simulink model "model_ROV_MPC_wLinFeed_NoTime"  (R2022b)
settings: Solver=VariableStepAuto  StartTime=0.0  StopTime=50  RelTol=1e-3
undefined symbols (not defined in the file): dt, magnitude, t0
libraries: realtime_pacer_lib x1, sim3dlib x1, uavsim3dlib x1
settings Model: Creator=anton  LastModifiedBy=anton

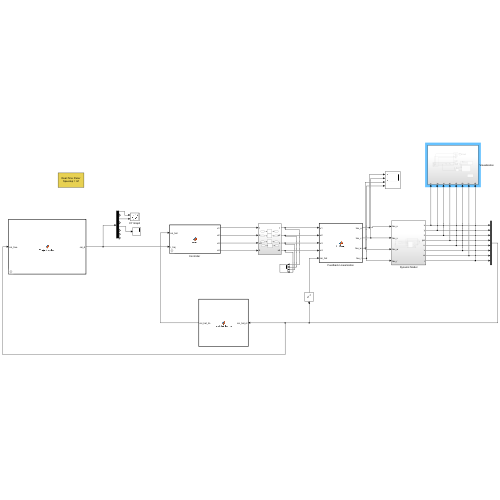
[thumbnail: Simulink's stored preview of the top-level diagram]
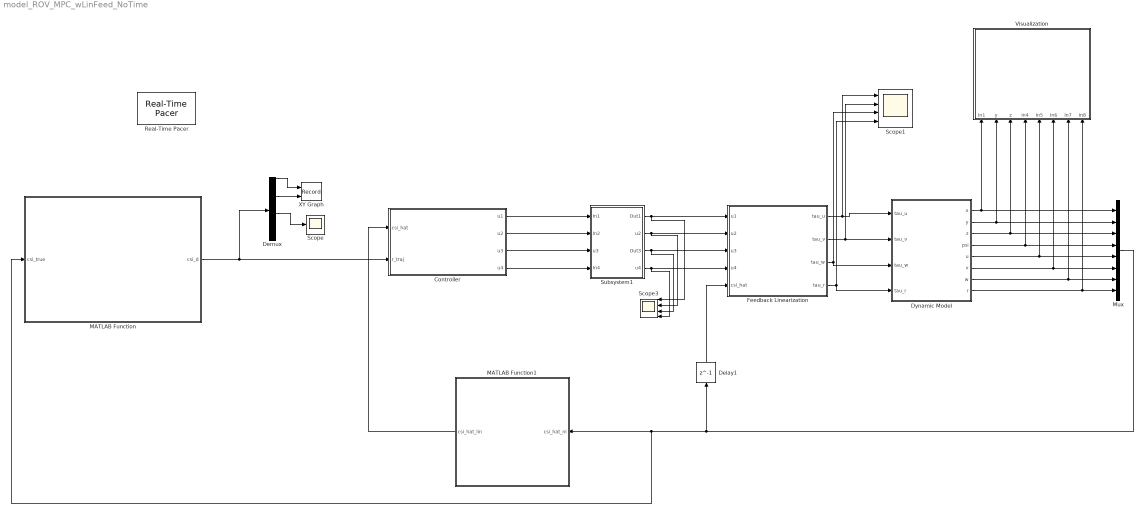
== system model_ROV_MPC_wLinFeed_NoTime ==
  "Controller " : MATLAB Function  TreatAsAtomicUnit=on  mask{dt=dt, t0=t0}
      mask prompts: dt "tempo di campionamento"; t0 "Start mission time"
  Delay1 : Delay  DelayLength=1  InitialCondition=[0 0 0 0 0 0 0 0]'  SampleTime=dt
  Demux : Demux  Outputs=8
  Dynamic Model : Subsystem
  Feedback Linearization : MATLAB Function  TreatAsAtomicUnit=on
  MATLAB Function : MATLAB Function  TreatAsAtomicUnit=on  mask{t0=t0}
      mask prompts: t0 "Tempo di partenza"
  MATLAB Function1 : MATLAB Function  TreatAsAtomicUnit=on
  Mux : Mux  Inputs=8
  Real-Time Pacer : realtime_pacer_lib/Real-Time Pacer  simTimePerRealTime=inf
  Scope : Scope
  Scope1 : Scope  NumInputPorts=4
  Scope3 : Scope  NumInputPorts=4
  Subsystem1 : Subsystem
  Visualization : Subsystem
  XY Graph : Record  FileSettingsInternal="{\"entries\":[{\"content\":{\"excelSettings\":{\"content\":{},\"type\":\"Streamout.ExcelSettings\"}},\"type\":\"Streamout.FileSettingStorage\",\"uuid\":\"\"}],\"packageUris\":[\"http:\\/\\/schema.mathworks.com\\/mf0\\/streamout_blocks\\/R2020a\"],\"version\":\"1.0\"}"  Layout=[1 1]  SignalsInternal="{\"entries\":[{\"content\":{\"signals\":[{\"content\":{\"blockPath\":[],\"channel\":[],\"dimensions\":[1,1],\"domain\":\"\",\"lineColor\":\"#a2142f\",\"plots\":[1],\"port\":1,\"sid\":[\"\"],\"signalID\":10914,\"signalName\":\"Demux:1\"},\"type\":\"RecordBlkView.Signal\",\"uuid\":\"\"},{\"content\":{\"blockPath\":[],\"channel\":[],\"dimensions\":[1,1],\"domain\":\"\",\"lineColor\":\"#139fff\",\"plots\":[1],\"port\":2,\"sid\":[\"\"],\"signalID\":10918,\"signalName\":\"Demux:3\"},\"type\":\"RecordBlkView.Signal\",\"uuid\":\"\"}]},\"type\":\"RecordBlkView.InputSignals\",\"uuid\":\"\"}],\"packageUris\":[\"http:\\/\\/schema.mathworks.com\\/mf0\\/streamout_blocks\\/R2020a\"],\"version\":\"1.0\"}"  VisualizationBindings="{\"xyplotplugin\":{\"info\":[{\"series\":[{\"bindingParametersList\":[{\"parameter\":\"X-Axis\",\"signalID\":10914,\"signalName\":\"Demux:1\"},{\"parameter\":\"Y-Axis\",\"signalID\":10918,\"signalName\":\"Demux:3\"}],\"seriesID\":62600}],\"subplotID\":1}]}}"  CompatibilityTag=XY
  wires:
  Subsystem1/2(u2) -> Feedback Linearization/2(u2), Scope3/2
  Subsystem1/3(Out3) -> Feedback Linearization/3(u3), Scope3/3
  Subsystem1/4(u4) -> Scope3/4, Feedback Linearization/4(u4)
  "Controller "/1(u1) -> Subsystem1/1(In1)
  "Controller "/2(u2) -> Subsystem1/2(In2)
  "Controller "/3(u3) -> Subsystem1/3(u3)
  "Controller "/4(u4) -> Subsystem1/4(In4)
  Subsystem1/1(Out1) -> Scope3/1, Feedback Linearization/1(u1)
  MATLAB Function1/1(csi_hat_lin) -> "Controller "/1(csi_hat)
  Dynamic Model/1(x) -> Mux/1, Visualization/1(In1)
  Dynamic Model/2(y) -> Mux/2, Visualization/2(y)
  Dynamic Model/3(z) -> Mux/3, Visualization/3(z)
  Dynamic Model/4(psi) -> Mux/4, Visualization/4(In4)
  Dynamic Model/5(u) -> Mux/5, Visualization/5(In5)
  Dynamic Model/6(v) -> Mux/6, Visualization/6(In6)
  Dynamic Model/7(w) -> Mux/7, Visualization/7(In7)
  Dynamic Model/8(r) -> Mux/8, Visualization/8(In8)
  Feedback Linearization/1(tau_u) -> Dynamic Model/1(tau_u), Scope1/1
  Feedback Linearization/2(tau_v) -> Scope1/2, Dynamic Model/2(tau_v)
  Feedback Linearization/3(tau_w) -> Dynamic Model/3(tau_w), Scope1/3
  Feedback Linearization/4(tau_r) -> Dynamic Model/4(tau_r), Scope1/4
  Mux/1 -> Delay1/1, MATLAB Function/1(csi_true), MATLAB Function1/1(csi_hat_nl)
  Delay1/1 -> Feedback Linearization/5(csi_hat)
  MATLAB Function/1(csi_d) -> Demux/1, "Controller "/2(r_traj)
  Demux/1 -> XY Graph/1
  Demux/3 -> XY Graph/2
  Demux/5 -> Scope/1

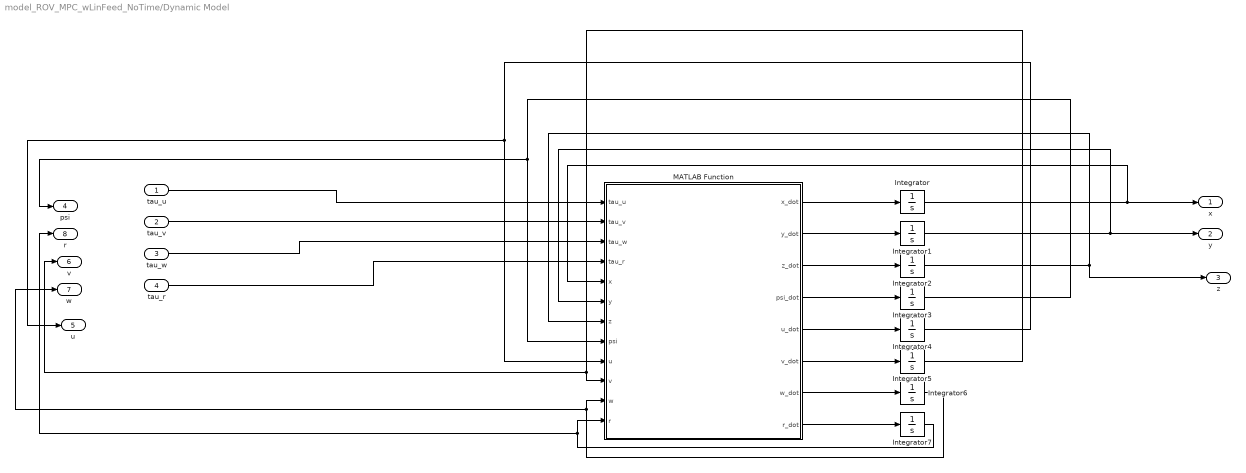
== system model_ROV_MPC_wLinFeed_NoTime/Dynamic Model ==
  tau_u : Inport
  tau_v : Inport  Port=2
  tau_w : Inport  Port=3
  tau_r : Inport  Port=4
  Integrator{,1..7} (8 alike) : Integrator
  MATLAB Function : MATLAB Function  TreatAsAtomicUnit=on
  x : Outport
  y : Outport  Port=2
  z : Outport  Port=3
  psi : Outport  Port=4
  u : Outport  Port=5
  v : Outport  Port=6
  w : Outport  Port=7
  r : Outport  Port=8
  wires:
  MATLAB Function/1(x_dot) -> Integrator/1
  Integrator3/1 -> psi/1, MATLAB Function/8(psi)
  MATLAB Function/6(v_dot) -> Integrator5/1
  MATLAB Function/4(psi_dot) -> Integrator3/1
  Integrator2/1 -> MATLAB Function/7(z), z/1
  Integrator4/1 -> u/1, MATLAB Function/9(u)
  Integrator6/1 -> w/1, MATLAB Function/11(w)
  Integrator7/1 -> r/1, MATLAB Function/12(r)
  MATLAB Function/5(u_dot) -> Integrator4/1
  MATLAB Function/7(w_dot) -> Integrator6/1
  tau_v/1 -> MATLAB Function/2(tau_v)
  MATLAB Function/8(r_dot) -> Integrator7/1
  tau_w/1 -> MATLAB Function/3(tau_w)
  MATLAB Function/3(z_dot) -> Integrator2/1
  Integrator1/1 -> y/1, MATLAB Function/6(y)
  Integrator5/1 -> v/1, MATLAB Function/10(v)
  tau_r/1 -> MATLAB Function/4(tau_r)
  Integrator/1 -> x/1, MATLAB Function/5(x)
  MATLAB Function/2(y_dot) -> Integrator1/1
  tau_u/1 -> MATLAB Function/1(tau_u)

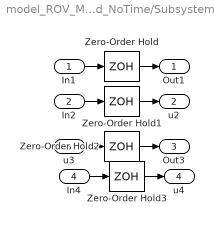
== system model_ROV_MPC_wLinFeed_NoTime/Subsystem1 ==
  In1 : Inport
  In2 : Inport  Port=2
  u3 : Inport  Port=3
  In4 : Inport  Port=4
  Zero-Order Hold{,1..3} (4 alike) : ZeroOrderHold  SampleTime=dt
  Out1 : Outport
  u2 : Outport  Port=2
  Out3 : Outport  Port=3
  u4 : Outport  Port=4
  wires:
  In1/1 -> Zero-Order Hold/1
  Zero-Order Hold/1 -> Out1/1
  In4/1 -> Zero-Order Hold3/1
  Zero-Order Hold1/1 -> u2/1
  Zero-Order Hold3/1 -> u4/1
  u3/1 -> Zero-Order Hold2/1
  In2/1 -> Zero-Order Hold1/1
  Zero-Order Hold2/1 -> Out3/1

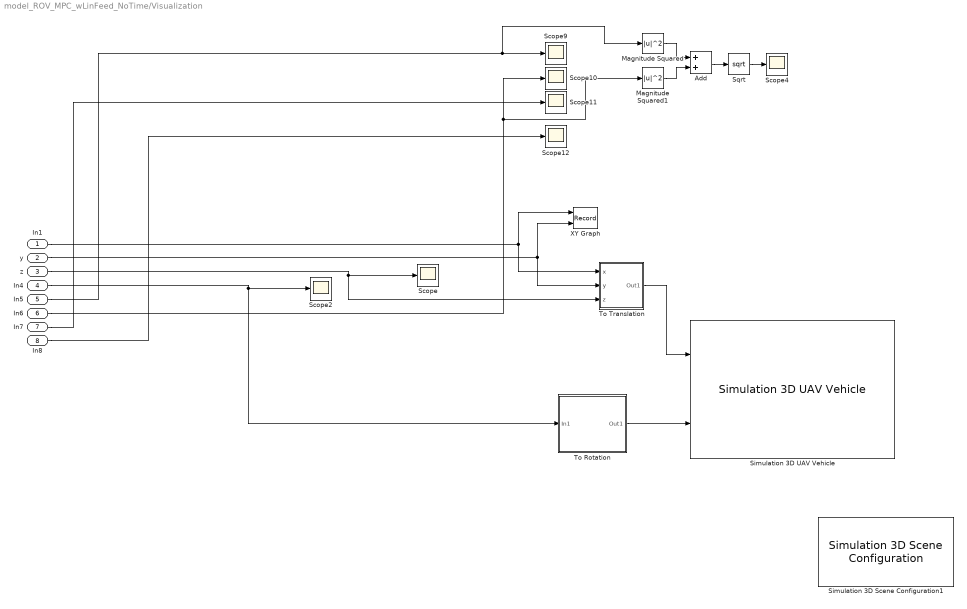
== system model_ROV_MPC_wLinFeed_NoTime/Visualization ==
  In1 : Inport
  y : Inport  Port=2
  z : Inport  Port=3
  In4 : Inport  Port=4
  In5 : Inport  Port=5
  In6 : Inport  Port=6
  In7 : Inport  Port=7
  In8 : Inport  Port=8
  Add : Sum
  Magnitude Squared : Math  Operator=magnitude^2
  Magnitude Squared1 : Math  Operator=magnitude^2
  Scope{,2,4,9..12} (7 alike) : Scope
  Simulation 3D Scene Configuration1 : sim3dlib/Simulation 3D Scene Configuration  Priority=0  ProjectFormat=Unreal Executable  SceneDesc=Empty scene  ProjectName=C:\Program Files\MATLAB\R2022b\toolbox\shared\sim3d_projects\automotive_project\UE4\WindowsNoEditor\VehicleSimulation.exe  ScenePath=/Game/Maps/HwStrght  EnableOpenDRIVE=off  vehTagList={'Scene Origin';'SimulinkVehicle1'}  vehTag=SimulinkVehicle1  OpVisEn=off  Ts=.02  EnableWindow=on  EnableRemoteAccess=off  EnableWeather=off  SunAltitude=40.0  SunAzimuth=90  clouds=10  wind=1  fog=0  rain=0  EnableGeospatial=off  OriginHeight=200  OriginLatitude=40.744652  OriginLongitude=-73.988864  MapStyle=Aerial  AdditionalAssetIDs=[]  UseAdvancedSunSky=off  SolarTime=11  TimeZone=-5  Day=21  Month=9  Year=2022  UseDaylightSavingTime=on  DSTStartDay=10  DSTStartMonth=3  DSTEndDay=3  DSTEndMonth=11  DSTSwitchHour=2  sensorTag=MainCamera2  sensorId=2  sensorName=MainCamera2  mountLoc=Origin  offsetFlag=off  tmountOffset=[0, 0, 0]  rmountOffset=[0, 0, 0]  HorizontalResolution=1280  VerticalResolution=720  HorizontalFOV=60  mountPoint=[0 0 0]  mountOrientation=[0 0 0]  aMode=5  ID=2  GeoTrigger=Inactive
      settings: LibrarySourceBlock=sl3dlib/Simulation 3D/Simulation 3D Scene Configuration
  Simulation 3D UAV Vehicle : uavsim3dlib/Simulation 3D UAV Vehicle  Priority=-1  Mesh=Fixed wing  MeshPath=C:\Users\angel\Downloads\bluerov2.dae  Color=Yellow  ActorName=SimulinkVehicle1  InitialTranslation=[0 0 0]  InitialRotation=[0 0 0]  SampleTime=-1  ActorType=SimulinkVehicle  ID=1  aMode=4  ActorTag=SimulinkVehicle1
  Sqrt : Sqrt
  To Rotation : Subsystem
  To Translation : Subsystem
  XY Graph : Record  FileSettingsInternal="{\"entries\":[{\"content\":{\"excelSettings\":{\"content\":{},\"type\":\"Streamout.ExcelSettings\"}},\"type\":\"Streamout.FileSettingStorage\",\"uuid\":\"\"}],\"packageUris\":[\"http:\\/\\/schema.mathworks.com\\/mf0\\/streamout_blocks\\/R2020a\"],\"version\":\"1.0\"}"  Layout=[1 1]  SignalsInternal="{\"entries\":[{\"content\":{\"signals\":[{\"content\":{\"blockPath\":[],\"channel\":[],\"dimensions\":[1,1],\"domain\":\"\",\"lineColor\":\"#0072bd\",\"plots\":[1],\"port\":1,\"sid\":[\"\"],\"signalID\":10906,\"signalName\":\"In1\"},\"type\":\"RecordBlkView.Signal\",\"uuid\":\"\"},{\"content\":{\"blockPath\":[],\"channel\":[],\"dimensions\":[1,1],\"domain\":\"\",\"lineColor\":\"#d95319\",\"plots\":[1],\"port\":2,\"sid\":[\"\"],\"signalID\":10910,\"signalName\":\"y\"},\"type\":\"RecordBlkView.Signal\",\"uuid\":\"\"}]},\"type\":\"RecordBlkView.InputSignals\",\"uuid\":\"\"}],\"packageUris\":[\"http:\\/\\/schema.mathworks.com\\/mf0\\/streamout_blocks\\/R2020a\"],\"version\":\"1.0\"}"  VisualizationBindings="{\"xyplotplugin\":{\"info\":[{\"series\":[{\"bindingParametersList\":[{\"parameter\":\"X-Axis\",\"signalID\":10906,\"signalName\":\"In1\"},{\"parameter\":\"Y-Axis\",\"signalID\":10910,\"signalName\":\"y\"}],\"seriesID\":32775}],\"subplotID\":1}]}}"  CompatibilityTag=XY
  wires:
  In5/1 -> Magnitude Squared/1, Scope9/1
  To Translation/1(Out1) -> Simulation 3D UAV Vehicle/1
  Add/1 -> Sqrt/1
  Sqrt/1 -> Scope4/1
  z/1 -> To Translation/3(z), Scope/1
  In6/1 -> Scope10/1, Magnitude Squared1/1
  In7/1 -> Scope11/1
  Magnitude Squared/1 -> Add/1
  To Rotation/1(Out1) -> Simulation 3D UAV Vehicle/2
  In1/1 -> To Translation/1(x), XY Graph/1
  Magnitude Squared1/1 -> Add/2
  y/1 -> XY Graph/2, To Translation/2(y)
  In8/1 -> Scope12/1
  In4/1 -> Scope2/1, To Rotation/1(In1)

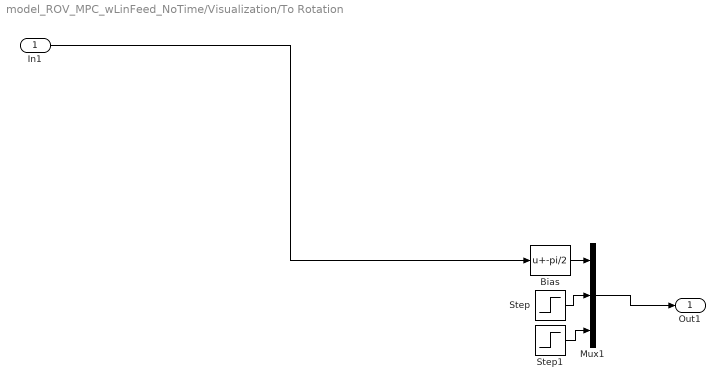
== system model_ROV_MPC_wLinFeed_NoTime/Visualization/To Rotation ==
  In1 : Inport
  Bias : Bias  Bias=-pi/2  SaturateOnIntegerOverflow=off
  Mux1 : Mux  Inputs=3
  Step : Step  After=0  SampleTime=0
  Step1 : Step  After=0  SampleTime=0
  Out1 : Outport
  wires:
  In1/1 -> Bias/1
  Step1/1 -> Mux1/3
  Step/1 -> Mux1/2
  Mux1/1 -> Out1/1
  Bias/1 -> Mux1/1

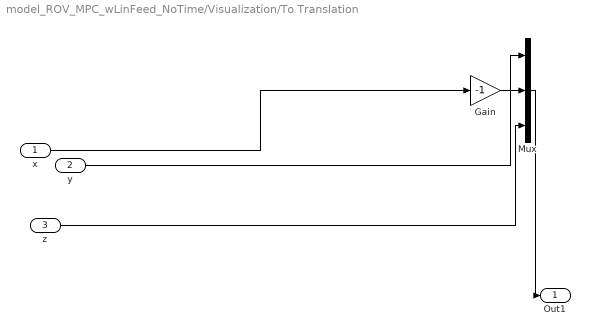
== system model_ROV_MPC_wLinFeed_NoTime/Visualization/To Translation ==
  x : Inport
  y : Inport  Port=2
  z : Inport  Port=3
  Gain : Gain  Gain=-1
  Mux : Mux  Inputs=3
  Out1 : Outport
  wires:
  Gain/1 -> Mux/2
  z/1 -> Mux/3
  x/1 -> Gain/1
  Mux/1 -> Out1/1
  y/1 -> Mux/1

== matlab function model_ROV_MPC_wLinFeed_NoTime/Feedback Linearization ==
  data: u1 input; tau_u output size=1; u2 input; u3 input; u4 input; csi_hat input; tau_v output size=1; tau_w output size=1; tau_r output size=1
function [tau_u,tau_v,tau_w,tau_r] = LinFeed(u1,u2,u3,u4,csi_hat)

psi = csi_hat(4);
u = csi_hat(5);
v = csi_hat(6);
w = csi_hat(7);
r = csi_hat(8);

m = 12;
d = 0.338;
l = 0.457;

I = 1/12*m*(d^2+l^2);

Y_v_dot = 0;
Y_r = 0;
X_u_dot = 0;
X_u = 0;
Y_v = 0;
Z_w = 0;
N_r = 0;
N_r_r = 0;

tau_u = (m*cos(psi)*(u1 + r*(v*cos(psi) + u*sin(psi)) - (cos(psi)*(X_u*u - r*(Y_r*r + Y_v_dot*v)))/m + (sin(psi)*(Y_v*v + X_u_dot*r*u))/m))/(cos(psi)^2 + sin(psi)^2) - (m*sin(psi)*(r*(u*cos(psi) - v*sin(psi)) - u2 + (sin(psi)*(X_u*u - r*(Y_r*r + Y_v_dot*v)))/m + (cos(psi)*(Y_v*v + X_u_dot*r*u))/m))/(cos(psi)^2 + sin(psi)^2);
tau_v =  - (m*sin(psi)*(u1 + r*(v*cos(psi) + u*sin(psi)) - (cos(psi)*(X_u*u - r*(Y_r*r + Y_v_dot*v)))/m + (sin(psi)*(Y_v*v + X_u_dot*r*u))/m))/(cos(psi)^2 + sin(psi)^2) - (m*cos(psi)*(r*(u*cos(psi) - v*sin(psi)) - u2 + (sin(psi)*(X_u*u - r*(Y_r*r + Y_v_dot*v)))/m + (cos(psi)*(Y_v*v + X_u_dot*r*u))/m))/(cos(psi)^2 + sin(psi)^2);
tau_w = m*(u3 - Z_w*w/m);
tau_r = I*(u4 - (u*(Y_r*r + Y_v_dot*v) + r*(N_r + N_r_r*r) - X_u_dot*u*v)/I);

== matlab function model_ROV_MPC_wLinFeed_NoTime/Dynamic Model/MATLAB Function ==
  data: tau_u input; tau_v input; tau_w input; tau_r input; x input; y input; z input; psi input; u input; x_dot output; v input; w input; r input; y_dot output; z_dot output; psi_dot output; u_dot output; v_dot output; w_dot output; r_dot output
function [x_dot,y_dot,z_dot,psi_dot,u_dot,v_dot,w_dot,r_dot] = Dynamics(tau_u,tau_v,tau_w,tau_r,x,y,z,psi,u,v,w,r)

m = 12;
d = 0.338;
l = 0.457;

I = 1/12*m*(d^2+l^2);

Y_v_dot = 0;
Y_r = 0;
X_u_dot = 0;
X_u = 0;
Y_v = 0;
Z_w = 0;
N_r = 0;
N_r_r = 0;


M = diag([m m m I]);
C = [0 0 0 Y_v_dot*v + Y_r*r;
     0 0 0 -X_u_dot*u;
     0 0 0 0;
     -Y_v_dot*v-Y_r*r X_u_dot*u 0 0];
D = diag([-X_u -Y_v -Z_w -N_r-N_r_r*r]);

ni = [u,v,w,r]';
tau = [tau_u,tau_v,tau_w,tau_r]';


ni_dot = inv(M)*(-C*ni - D*ni + tau);

eta_dot = [cos(psi) -sin(psi) 0 0;
           sin(psi) cos(psi) 0 0;
           0 0 1 0;
           0 0 0 1]*ni;

x_dot = eta_dot(1);
y_dot = eta_dot(2);
z_dot = eta_dot(3);
psi_dot = eta_dot(4);

u_dot = ni_dot(1);
v_dot = ni_dot(2);
w_dot = ni_dot(3);
r_dot = ni_dot(4);

== matlab function model_ROV_MPC_wLinFeed_NoTime/MATLAB Function ==
  data: csi_d output size=[8,1]; csi_true input size=[8,1]; t0 parameter
function csi_d  = TrajectoryTest(csi_true,t0)
    x = [];
    y = [];
    z = [];
    x_true = csi_true(1);
    y_true = csi_true(2);
    z_true = csi_true(3);
    psi = [];


    %% INTERPOLAZIONE CON SPLINE CUBICHE
    % Punti di Interpolazione
    x1 = 0;
    y1 = 0;
    z1 = 2;
    x2 = 10;
    y2 = 5;
    z2 = 2;
    x3 = 15;
    y3 = 0;
    z3 = 4;
    J_eval = [];
    r = [];
    
    coeff_acc = 5;
    coeff_vel = 5;
    coeff_temp = 1;

    % MINIMIZZAZIONE DEL COSTO
    
    i=[0.1:0.1:100];
    for h = i
        J = 2*coeff_temp*h + (3*coeff_acc*(x1^2 - 4*x1*x2 + 2*x1*x3 + 4*x2^2 - ...
            4*x2*x3 + x3^2 + y1^2 - 4*y1*y2 + 2*y1*y3 + 4*y2^2 - 4*y2*y3 + y3^2 +...
        z1^2 - 4*z1*z2 + 2*z1*z3 + 4*z2^2 - 4*z2*z3 + z3^2))/(2*h^3) +...
        (coeff_vel*(11*x1^2 - 24*x1*x2 + 2*x1*x3 + 24*x2^2 - 24*x2*x3 + 11*x3^2 + ...
        11*y1^2 - 24*y1*y2 + 2*y1*y3 + 24*y2^2 - 24*y2*y3 + 11*y3^2 + 11*z1^2 - ...
        24*z1*z2 + 2*z1*z3 + 24*z2^2 - 24*z2*z3 + 11*z3^2))/(10*h) +...
        (coeff_vel*(13*x1^2 - 36*x1*x2 + 10*x1*x3 + 36*x2^2 - 36*x2*x3 + ...
        13*x3^2 + 13*y1^2 - 36*y1*y2 + 10*y1*y3 + 36*y2^2 - 36*y2*y3 + ...
        13*y3^2 + 13*z1^2 - 36*z1*z2 + 10*z1*z3 + 36*z2^2 - 36*z2*z3 + 13*z3^2))/(8*h^2);
        J_eval = [J_eval,J];
    end

    [J_min,i_min] = (min(J_eval));
    h_ottimo = (i(i_min))

    % Spline sulla x
    Mx = 3/(2*h_ottimo^2)*(x1+x3-2*x2);
    
    bx1 = 0;
    bx2 = Mx/2;
    dx1 = x1;
    dx2 = x2;
    ax1 = Mx/(6*h_ottimo);
    ax2 = -Mx/(6*h_ottimo);
    cx1 = (x2-x1)/h_ottimo - Mx*h_ottimo/6;
    cx2 = (x3-x2)/h_ottimo - Mx*h_ottimo/3;
    
    % Spline sulla y
    My = 3/(2*h_ottimo^2)*(y1+y3-2*y2);
    
    by1 = 0;
    by2 = My/2;
    dy1 = y1;
    dy2 = y2;
    ay1 = My/(6*h_ottimo);
    ay2 = -My/(6*h_ottimo);
    cy1 = (y2-y1)/h_ottimo - My*h_ottimo/6;
    cy2 = (y3-y2)/h_ottimo - My*h_ottimo/3;
    
    % Spline sulla z
    Mz = 3/(2*h_ottimo^2)*(z1+z3-2*z2);
    
    bz1 = 0;
    bz2 = Mz/2;
    dz1 = z1;
    dz2 = z2;
    az1 = Mz/(6*h_ottimo);
    az2 = -Mz/(6*h_ottimo);
    cz1 = (z2-z1)/h_ottimo - Mz*h_ottimo/6;
    cz2 = (z3-z2)/h_ottimo - Mz*h_ottimo/3;


    for t=t0:h_ottimo/149:t0+h_ottimo
        x = [x,ax1*(t-t0)^3 + bx1*(t-t0)^2 + cx1*(t-t0) + dx1];
        y = [y,ay1*(t-t0)^3 + by1*(t-t0)^2 + cy1*(t-t0) + dy1];
        z = [z,az1*(t-t0)^3 + bz1*(t-t0)^2 + cz1*(t-t0) + dz1];
        psi = [psi,atan2(3*ay1*(t-t0)^2 + 2*by1*(t-t0) + cy1,3*ax1*(t-t0)^2 + 2*bx1*(t-t0) + cx1)];
    end
    for t=t0+h_ottimo:h_ottimo/149:t0+2*h_ottimo
        x = [x,ax2*(t-t0-h_ottimo)^3 + bx2*(t-t0-h_ottimo)^2 + cx2*(t-t0-h_ottimo) + dx2];
        y = [y,ay2*(t-t0-h_ottimo)^3 + by2*(t-t0-h_ottimo)^2 + cy2*(t-t0-h_ottimo) + dy2];
        z = [z,az2*(t-t0-h_ottimo)^3 + bz2*(t-t0-h_ottimo)^2 + cz2*(t-t0-h_ottimo) + dz2];
        psi = [psi,atan2(3*ay2*(t-t0-h_ottimo)^2 + 2*by2*(t-t0-h_ottimo) + cy2,3*ax2*(t-t0-h_ottimo)^2 + 2*bx2*(t-t0-h_ottimo) + cx2)];
    end
    
    e = vecnorm([x_true;y_true;z_true]*ones(1,300) - [x;y;z]);

    [~,i] = min(e);

    csi_d_dot = [cos(psi(i)) -sin(psi(i)) 0 0;
                 sin(psi(i)) cos(psi(i)) 0 0;
                 0 0 1 0;
                 0 0 0 1]*[0.5;0;0;0];

    csi_d = [x(i),csi_d_dot(1),y(i),csi_d_dot(2),z(i),csi_d_dot(3),psi(i),csi_d_dot(4)]';
    
end

== matlab function model_ROV_MPC_wLinFeed_NoTime/Controller  ==
  data: u1 output; csi_hat input; r_traj input; u2 output; u3 output; u4 output; dt parameter
function [u1,u2,u3,u4] = MPC(csi_hat,r_traj,dt)
% in tempo discreto
A = dt*blkdiag([0 1;0 0],[0 1;0 0],[0 1;0 0],[0 1;0 0]) + eye(8,8);
B = dt*blkdiag([0;1],[0;1],[0;1],[0;1]);
C = blkdiag([1 0;0 1],[1 0;0 1],[1 0;0 1],[1 0;0 1]);
Np = 4;
Nc = 4;
Zero = zeros(8,4);
PHI = [C*B Zero Zero Zero ; 
        C*A*B C*B Zero Zero; 
        C*A^2*B C*A*B C*B Zero; 
        C*A^3*B C*A^2*B C*A*B C*B];
F = [C*A; 
    C*A^2; 
    C*A^3; 
    C*A^4];
% 
% Np = 10; % orizzonte di predizione
% Nc = 5; % orizzonte di controllo, numero di comandi con cui facciamo predizione
% Zero = zeros(4,4);
% 
% PHI = [C*B Zero Zero Zero Zero; 
%         C*A*B C*B Zero Zero Zero; 
%         C*A^2*B C*A*B C*B Zero Zero; 
%         C*A^3*B C*A^2*B C*A*B C*B Zero;
%         C*A^4*B C*A^3*B C*A^2*B C*A*B C*B;
%         C*A^5*B C*A^4*B C*A^3*B C*A^2*B C*A*B;
%         C*A^6*B C*A^5*B C*A^4*B C*A^3*B C*A^2*B;
%         C*A^7*B C*A^6*B C*A^5*B C*A^4*B C*A^3*B;
%         C*A^8*B C*A^7*B C*A^6*B C*A^5*B C*A^4*B;
%         C*A^9*B C*A^8*B C*A^7*B C*A^6*B C*A^5*B];
% F = [C*A; 
%     C*A^2; 
%     C*A^3; 
%     C*A^4;
%     C*A^5; 
%     C*A^6; 
%     C*A^7;
%     C*A^8; 
%     C*A^9; 
%     C*A^10];
% 
 Rc = 0.05*eye(4*(Nc));

% x_d = 1;
% y_d = 1;
% z_d = 1;
% psi_d = pi/2; 

%% INTERPOLAZIONE POLINOMIALE

% x0 = 0;
% y0 = 0;
% t0 = 0;
% x1 = 2;
% y1 = 5;
% t1 = 30;
% x2 = 4;
% y2 = 0;
% t2 = 60;
% z0 = 0;
% z1 = 3;
% z2 = 0;
% r = [];
% 
% for i=1:Np
%     t = clk + i*dt;
%     L0 = (t-t1)/(t0-t1) * (t-t2)/(t0-t2);
%     L1 = (t-t0)/(t1-t0) * (t-t2)/(t1-t2);
%     L2 = (t-t0)/(t2-t0) * (t-t1)/(t2-t1);
%     x_d = x0*L0 + x1*L1 + x2*L2;
%     y_d = y0*L0 + y1*L1 + y2*L2;
%     z_d = z0*L0 + z1*L1 + z2*L2;
% 
%     x_d_dot = (x0 - x2)/(t0 - t2) - ((x0 - x1)*(t0 - 2*t + t2))/((t0 - t1)*(t0 - t2)) + ((x1 - x2)*(t0 - 2*t + t2))/((t0 - t2)*(t1 - t2));
%     y_d_dot = (y0 - y2)/(t0 - t2) - ((y0 - y1)*(t0 - 2*t + t2))/((t0 - t1)*(t0 - t2)) + ((y1 - y2)*(t0 - 2*t + t2))/((t0 - t2)*(t1 - t2));
%     psi_d = atan2(y_d_dot,x_d_dot);
%     
%     if(t==t2)
%         psi_2 = psi_d;
%     end
%     if t>=t2
%         r = [r;x2;y2;z2;psi_2];
%     else
%         r = [r;x_d;y_d;z_d;psi_d];
%     end
% end

% csi_d = [p_x p_y p_z psi_d]';
% csi_d_dot = [v_x v_y v_z psi_d_dot]';
% csi_d_2dot = [acc_x acc_y acc_z psi_d_2dot]';


%% Calcolo del controllo

% Rs = [eye(4,4);
%     eye(4,4);
%     eye(4,4);
%     eye(4,4);
%     eye(4,4);
%     eye(4,4);
%     eye(4,4);
%     eye(4,4);
%     eye(4,4);
%     eye(4,4)];

r = [r_traj;r_traj;r_traj;r_traj];

% DeltaU = ((PHI'*PHI + Rc)^-1*PHI'*(Rs*r_k - F*csi_hat));
DeltaU = ((PHI'*PHI + Rc)^-1*PHI'*(r - F*csi_hat));
u_k = DeltaU(1:4); %+ u_kmeno1;
u1 = u_k(1);
u2 = u_k(2);
u3 = u_k(3);
u4 = u_k(4);

end

== matlab function model_ROV_MPC_wLinFeed_NoTime/MATLAB Function1 ==
  data: csi_hat_nl input size=[8,1]; csi_hat_lin output size=[8,1]
function csi_hat_lin = VariableTrans(csi_hat_nl)

    x = csi_hat_nl(1);
    y = csi_hat_nl(2);
    z = csi_hat_nl(3);
    psi = csi_hat_nl(4);
    x_dot = csi_hat_nl(5)*cos(csi_hat_nl(4)) - csi_hat_nl(6)*sin(csi_hat_nl(4));
    y_dot = csi_hat_nl(5)*sin(csi_hat_nl(4)) + csi_hat_nl(6)*cos(csi_hat_nl(4));
    z_dot = csi_hat_nl(7);
    psi_dot = csi_hat_nl(8);

    csi_hat_lin = [x  x_dot y y_dot z z_dot psi psi_dot]';
